simulink library "coros_protocol_lib"  (R2021a)
settings: Solver=VariableStepAuto  StartTime=0.0  StopTime=10.0  RelTol=1e-3
libraries: robotlib x3, $bdroot x2
settings Model: Creator=MyPC  LastModifiedBy=MyPC

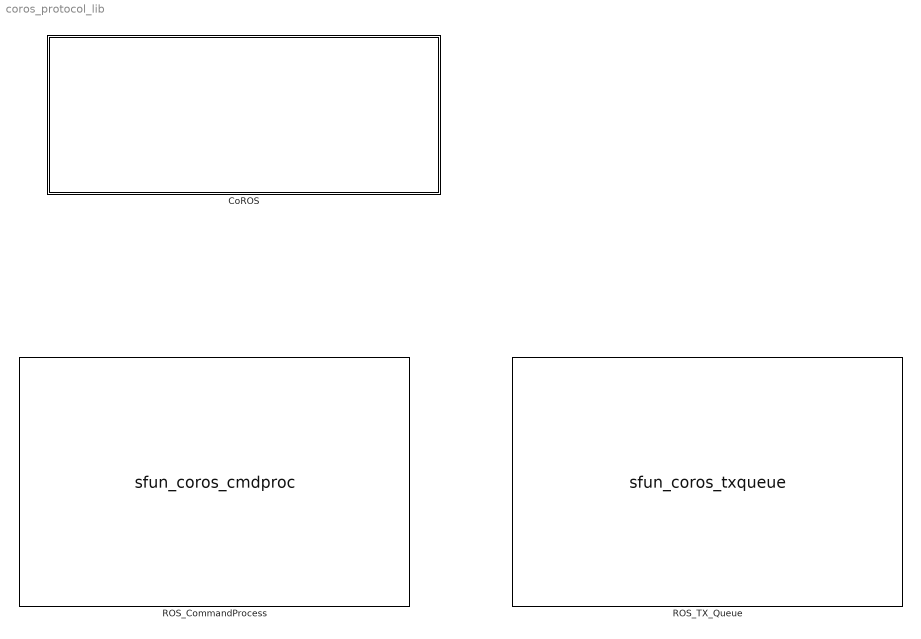
== system coros_protocol_lib ==
  CoROS : Subsystem  TreatAsAtomicUnit=on
      mask Display:
      | text(0.5, 0.5, '\bf\it\color[rgb]{0,0.5,0.5}\fontsize{40} CoROS', 'horizontalAlignment', 'center', 'texmode', 'on')
      | text(0.5, 0.3, '\bf\it\color[rgb]{0.5,0.5,0.5}\fontsize{15} Calibration on ROS', 'horizontalAlignment', 'center', 'texmode', 'on')
  ROS_CommandProcess : S-Function  FunctionName=sfun_coros_cmdproc  SFunctionDeploymentMode=off  EnableBusSupport=off  mask(CoROS_CmdProc){}
      mask help:
      | This block implements CoROS (Calibration on ROS) protocol.
      | When placed in a ROS based model, it collect the variables and generate code to implement the PC to ROS-ECU interactive communication.
      mask Display:
      | color('cyan')
      | port_label('input',1,'Command ID');
      | port_label('input',2,'Command String');
      | port_label('input',3,'_cmd_string_size');
      | port_label('input',4,'Command Options');
      | port_label('input',5,'Payload Data');
      | port_label('input',6,'_payload_size');
      | port_label('input',7,'_orig_payload_size');
      | 
      | text(0.5,0.5,'\fontsize{20} CoROS Protocol','horizontalAlignment', 'center', 'texmode','on')
  ROS_TX_Queue : S-Function  FunctionName=sfun_coros_txqueue  SFunctionDeploymentMode=off  EnableBusSupport=off  mask(CoROS Tx Queue){}
      mask help:
      | This block is part of the CoROS (Calibration on ROS) protocol, should be used in combination with the CoROS CmdProc block.
      | When placed in a ROS based model, it maintains a FIFO Tx queue that transmits response packets (incl. DAQ) when executed.
      | This block intends to be connected with a Function-Call subsystem downstream that contains a ROS Publish block, it calls the subsystem iteratively "while" the queue is not empty, thus to transmit all the messages in one time step. Note that the "Queue size" of the ROS Publish block should be adapted with the queue size of this block.
      mask Display:
      | color('cyan')
      | port_label('output',1,'Tx FcnCall()');
      | port_label('output',2,'Response ID');
      | port_label('output',3,'Response String');
      | port_label('output',4,'_resp_str_size');
      | port_label('output',5,'Response Options');
      | port_label('output',6,'Payload Data');
      | port_label('output',7,'_payload_size');
      | 
      | text(0.5,0.5,'\fontsize{20} CoROS Tx Queue','horizontalAlignment', 'center', 'texmode','on')

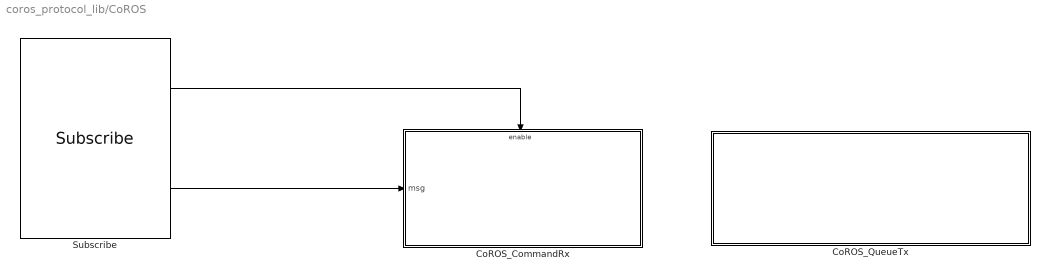
== system coros_protocol_lib/CoROS ==
  CoROS_CommandRx : Subsystem
  CoROS_QueueTx : Subsystem
  Subscribe : robotlib/Subscribe  topicSource=Specify your own  topic=/coros_cal  messageType=coros_msgs/cmdpacket  SampleTime=-1  legacyBusStruct=off  messageQueueLength=5
  wires:
  Subscribe/1 -> CoROS_CommandRx/Enable
  Subscribe/2 -> CoROS_CommandRx/1(msg)

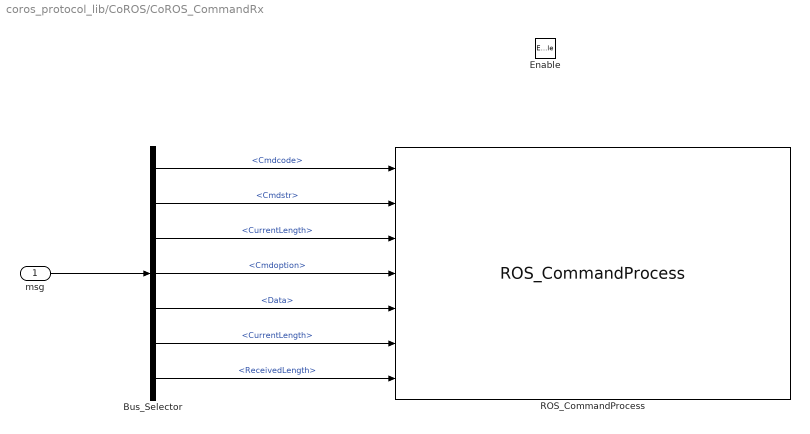
== system coros_protocol_lib/CoROS/CoROS_CommandRx ==
  msg : Inport
  Enable : EnablePort
  Bus_Selector : BusSelector  OutputSignals=Cmdcode,Cmdstr,Cmdstr_SL_Info.CurrentLength,Cmdoption,Data,Data_SL_Info.CurrentLength,Data_SL_Info.ReceivedLength
  ROS_CommandProcess : $bdroot/ROS_CommandProcess
  wires:
  msg/1 -> Bus_Selector/1
  Bus_Selector/2 -> ROS_CommandProcess/2  "<Cmdstr>"
  Bus_Selector/1 -> ROS_CommandProcess/1  "<Cmdcode>"
  Bus_Selector/3 -> ROS_CommandProcess/3  "<CurrentLength>"
  Bus_Selector/4 -> ROS_CommandProcess/4  "<Cmdoption>"
  Bus_Selector/5 -> ROS_CommandProcess/5  "<Data>"
  Bus_Selector/6 -> ROS_CommandProcess/6  "<CurrentLength>"
  Bus_Selector/7 -> ROS_CommandProcess/7  "<ReceivedLength>"

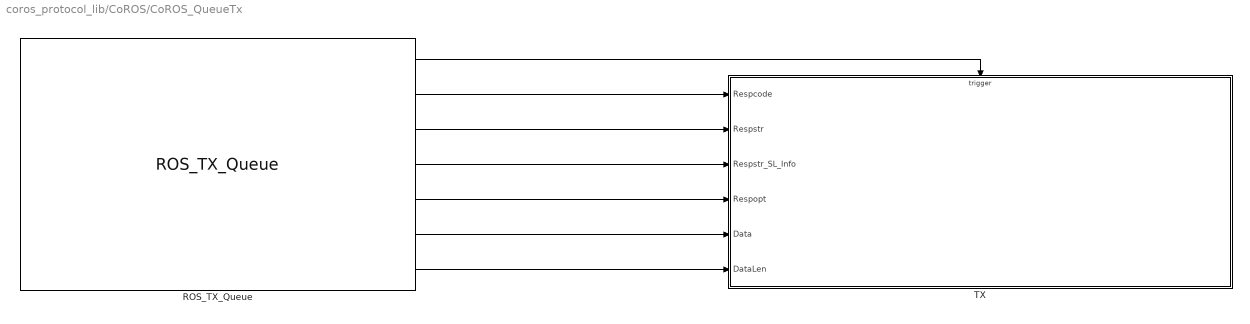
== system coros_protocol_lib/CoROS/CoROS_QueueTx ==
  ROS_TX_Queue : $bdroot/ROS_TX_Queue
  TX : Subsystem
  wires:
  ROS_TX_Queue/1 -> TX/Trigger
  ROS_TX_Queue/2 -> TX/1(Respcode)
  ROS_TX_Queue/3 -> TX/2(Respstr)
  ROS_TX_Queue/4 -> TX/3(Respstr_SL_Info)
  ROS_TX_Queue/5 -> TX/4(Respopt)
  ROS_TX_Queue/6 -> TX/5(Data)
  ROS_TX_Queue/7 -> TX/6(DataLen)

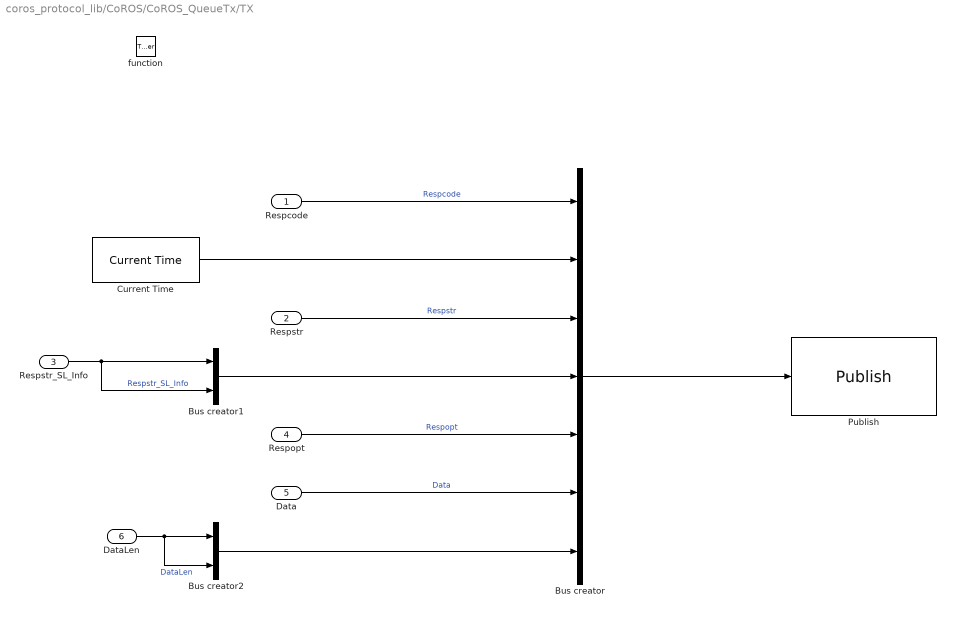
== system coros_protocol_lib/CoROS/CoROS_QueueTx/TX ==
  Respcode : Inport
  Respstr : Inport  Port=2
  Respstr_SL_Info : Inport  Port=3
  Respopt : Inport  Port=4
  Data : Inport  Port=5
  DataLen : Inport  Port=6
  function : TriggerPort  TriggerType=function-call  VariantControl=(inherit)
  Bus creator : BusCreator  Inputs=7  OutDataTypeStr=Bus: SL_Bus_coros_protocol_lib_coros_msgs_resppacket  NonVirtualBus=on
      settings: AttributesFormatString=CopyFcn  CopyFcn=set_param(gcb, 'OutDataTypeStr', sprintf('Bus: SL_Bus_%s_coros_msgs_resppacket', bdroot(gcb)));  InheritFromInputs=off
  Bus creator1 : BusCreator  Inputs=2
  Bus creator2 : BusCreator  Inputs=2
  Current Time : robotlib/Current Time  OutputFormat=bus  SampleTime=-1  ModelName=test_sendrcv
      settings: SourceProductBaseCode=RR
  Publish : robotlib/Publish  topicSource=Specify your own  topic=/coros_resp  messageType=coros_msgs/resppacket  legacyBusStruct=off  messageQueueLength=50
  wires:
  Bus creator/1 -> Publish/1
  Respcode/1 -> Bus creator/1  "Respcode"
  Current Time/1 -> Bus creator/2
  Respstr/1 -> Bus creator/3  "Respstr"
  Data/1 -> Bus creator/6  "Data"
  Respopt/1 -> Bus creator/5  "Respopt"
  Bus creator1/1 -> Bus creator/4
  Respstr_SL_Info/1 -> Bus creator1/2, Bus creator1/1  "Respstr_SL_Info"
  DataLen/1 -> Bus creator2/2, Bus creator2/1  "DataLen"
  Bus creator2/1 -> Bus creator/7
